simulink model "s0224"  (Simulink 6.0)
settings: Solver=ode3  SolverMode=SingleTasking  StartTime=0.0  StopTime=900  FixedStep=1  MaxStep=1  RelTol=1e-3  AbsTol=1e-6
values from neighbouring files (symbols this model uses):
  Dudach = 0    [m0221d.m]    (also in m0224.m = DudachVec(i))
libraries: simulink x1
settings Model: LastModifiedBy=Froriep
settings DataIOCC: LimitDataPoints=off  SaveOutput=off  SaveTime=off
settings OptimizationCC: BooleanDataType=off
settings DebuggingCC: SolverPrmCheckMsg=none
settings HardwareCC: TargetUnknown=on
settings GRTTargetCC: ModelReferenceCompliant=off  MatFileLogging=off

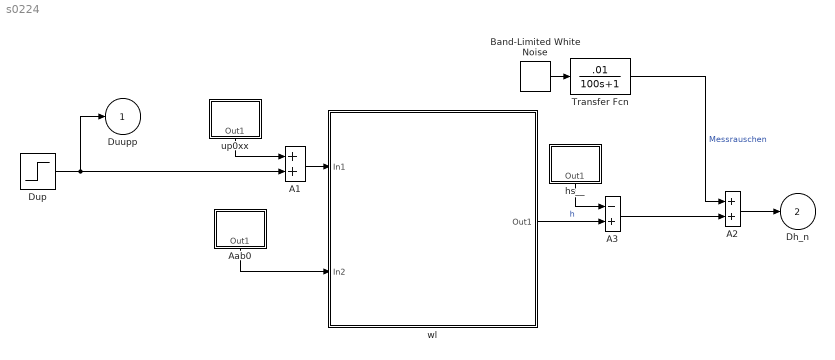
== system s0224 ==
  A1 : Sum  SaturateOnIntegerOverflow=on  InputSameDT=on
  A2 : Sum  SaturateOnIntegerOverflow=on  InputSameDT=on
  A3 : Sum  Inputs=-+  SaturateOnIntegerOverflow=on  InputSameDT=on
  Aab0 : Subsystem  Orientation=down  mask(Konstante){@1=Aab0}
      mask prompts: @1 "Wert"
      mask help: Konstante
      mask init:
      | Konst=@1;
      mask Display: disp('Aab0')
  Band-Limited White Noise : simulink/Sources/Band-Limited White Noise  Cov=[0.1]  Ts=1  seed=[23341]
  Dup : Step  After=Dudach  SampleTime=0
  Transfer Fcn : TransferFcn  Numerator=[.01]  Denominator=[100 1]
  hs__ : Subsystem  Orientation=down  mask(Konstante){@1=hs}
      mask prompts: @1 "Wert"
      mask help: Konstante
      mask init:
      | Konst=@1;
      mask Display: disp('hs')
  up0xx : Subsystem  Orientation=down  mask(Konstante){@1=up0}
      mask prompts: @1 "Wert"
      mask help: Konstante
      mask init:
      | Konst=@1;
      mask Display: disp('up0')
  wl : Subsystem
      mask Display: disp('Nichtlineares\nFüllstandsmodell')
  Duupp : Outport
  Dh_n : Outport  Port=2
  wires:
  Aab0/1(Out1) -> wl/2(In2)
  up0xx/1(Out1) -> A1/1
  hs__/1(Out1) -> A3/1
  A1/1 -> wl/1(In1)
  Dup/1 -> Duupp/1, A1/2
  wl/1(Out1) -> A3/2  "h"
  A3/1 -> A2/2
  A2/1 -> Dh_n/1
  Band-Limited White Noise/1 -> Transfer Fcn/1
  Transfer Fcn/1 -> A2/1  "Messrauschen"

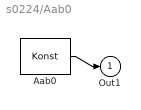
== system s0224/Aab0 ==
  Aab0 : Constant  Value=Konst
  Out1 : Outport
  wires:
  Aab0/1 -> Out1/1

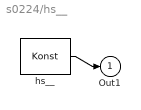
== system s0224/hs__ ==
  hs__ : Constant  Value=Konst
  Out1 : Outport
  wires:
  hs__/1 -> Out1/1

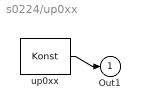
== system s0224/up0xx ==
  up0xx : Constant  Value=Konst
  Out1 : Outport
  wires:
  up0xx/1 -> Out1/1

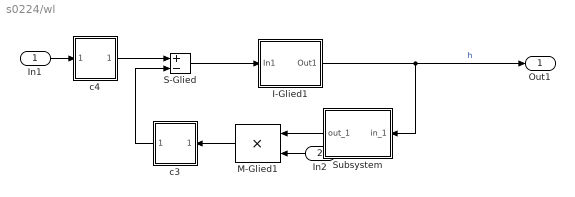
== system s0224/wl ==
  In1 : Inport  Port=1  LatchInput=off
  In2 : Inport  Orientation=left  Port=2  LatchInput=off
  I-Glied1 : Subsystem  mask(I-Glied){@1=hs}
      mask prompts: @1 "Anfangswert"
      mask help: I-Glied
      mask init:
      | x0=@1;
      mask Display: disp('I-Glied')
  M-Glied1 : Product  Orientation=left  SaturateOnIntegerOverflow=on  RndMeth=Zero  InputSameDT=on
  S-Glied : Sum  Inputs=+-  SaturateOnIntegerOverflow=on  InputSameDT=on
  Subsystem : Subsystem  Orientation=left
      mask Display: disp('Wurzel')
  c3 : Subsystem  Orientation=left  mask(P-Glied){@1=c1}
      mask prompts: @1 "Beiwert"
      mask help: P-Glied
      mask init:
      | Kp=@1;
      mask Display: disp('c1')
  c4 : Subsystem  mask(P-Glied){@1=c2}
      mask prompts: @1 "Beiwert"
      mask help: P-Glied
      mask init:
      | Kp=@1;
      mask Display: disp('c2')
  Out1 : Outport
  wires:
  I-Glied1/1(Out1) -> Subsystem/1(in_1), Out1/1  "h"
  c3/1(Out1) -> S-Glied/2
  Subsystem/1(out_1) -> M-Glied1/1
  M-Glied1/1 -> c3/1(In1)
  S-Glied/1 -> I-Glied1/1(In1)
  c4/1(Out1) -> S-Glied/1
  In1/1 -> c4/1(In1)
  In2/1 -> M-Glied1/2

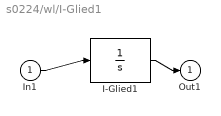
== system s0224/wl/I-Glied1 ==
  In1 : Inport  Port=1  LatchInput=off
  I-Glied1 : Integrator  InitialCondition=x0
  Out1 : Outport
  wires:
  In1/1 -> I-Glied1/1
  I-Glied1/1 -> Out1/1

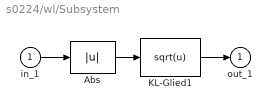
== system s0224/wl/Subsystem ==
  in_1 : Inport  Port=1  LatchInput=off
  Abs : Abs  SaturateOnIntegerOverflow=on
  KL-Glied1 : Fcn  Expr=sqrt(u)
  out_1 : Outport
  wires:
  KL-Glied1/1 -> out_1/1
  in_1/1 -> Abs/1
  Abs/1 -> KL-Glied1/1

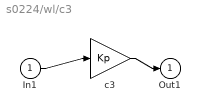
== system s0224/wl/c3 ==
  In1 : Inport  Port=1  LatchInput=off
  c3 : Gain  Gain=Kp  SaturateOnIntegerOverflow=on
  Out1 : Outport
  wires:
  In1/1 -> c3/1
  c3/1 -> Out1/1

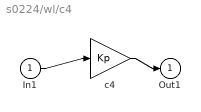
== system s0224/wl/c4 ==
  In1 : Inport  Port=1  LatchInput=off
  c4 : Gain  Gain=Kp  SaturateOnIntegerOverflow=on
  Out1 : Outport
  wires:
  In1/1 -> c4/1
  c4/1 -> Out1/1
